simulink model "saturn_ib_stack_test"  (Simulink 6.2)
settings: Solver=ode4  SolverMode=SingleTasking  StartTime=-20.0  StopTime=620  FixedStep=0.005  RelTol=1e-3
values from neighbouring files (symbols this model uses):
  A_z_deg = 82.8200    (= 82.82)    [AS205_presettings.m]
  BN_1_sec = 14.4    [AS205_presettings.m]
  DeltaV_b_mps = 7.2381    [AS205_presettings.m]
  epsilon_2_sec = 15.0    (= 15)    [AS205_presettings.m]
  epsilon_prime_sec = 3.0    (= 3)    [AS205_presettings.m]
  i_deg = 28.89597    [AS205_presettings.m]
  lambda_0_deg = 102.32900    (= 102.329)    [AS205_presettings.m]
  lambda_L_deg = -80.561141    [AS205_presettings.m]
  pad_roll_L_deg = 100.0    (= 100)    [AS205_presettings.m]
  phi_L_deg = 28.521963    [AS205_presettings.m]
  phi_L_prime_deg = 28.360795    [AS205_presettings.m]
  R_L_m = 6373385.0    (= 6373385)    [AS205_presettings.m]
  R_T_m = 6570774.0    (= 6570774)    [AS205_presettings.m]
  T3_FM_sec = 6.08    [AS205_presettings.m]
  T_HSL_sec = 5.0    (= 5)    [AS205_presettings.m]
  Theta_T_deg = 0.000    (= 0)    [AS205_presettings.m]
  V_T_mps = 7780.976    [AS205_presettings.m]
  Xdotdot_VGT_mps2 = -9.251    [AS205_presettings.m]
undefined symbols (not defined in the file or in its folder): e0_0, e1_0, e2_0, e3_0, m, s
libraries: simulink x99, aerolibconvert x83, aerolibutil x63, aerolibtransform2 x34, aerolibasang x2, aerolibatmos2 x2, aerolib6dofsys x2
(part 5 of 7)

== system saturn_ib_stack_test/Saturn_IB_Stack/S-IVB Stage/APS III Module/APS Thruster II ==
  Fire : Inport  Port=1  LatchInput=off
  Cg_m : Inport  Port=2  PortDimensions=3  LatchInput=off
  3x3 Cross Product : aerolibutil/3x3 Cross Product
  Add : Sum  Inputs=+-  OutScaling=2^-10
  Constant2 : Constant  Value=[0.0 0.0 0.0]
  Installation location (m) : Constant  Value=r_m  OutDataTypeMode=double
  Switch : Switch  Criteria=u2 ~= 0
  Thruster Force : Constant  Value=F_N  OutDataTypeMode=double
  F_N : Outport
  M_Nm : Outport  Port=2
  wires:
  Cg_m/1 -> Add/2
  Installation location (m)/1 -> Add/1
  Add/1 -> 3x3 Cross Product/1
  3x3 Cross Product/1 -> M_Nm/1
  Switch/1 -> 3x3 Cross Product/2, F_N/1
  Thruster Force/1 -> Switch/1
  Constant2/1 -> Switch/3
  Fire/1 -> Switch/2

== system saturn_ib_stack_test/Saturn_IB_Stack/S-IVB Stage/APS III Module/APS Thruster IV ==
  Fire : Inport  Port=1  LatchInput=off
  Cg_m : Inport  Port=2  PortDimensions=3  LatchInput=off
  3x3 Cross Product : aerolibutil/3x3 Cross Product
  Add : Sum  Inputs=+-  OutScaling=2^-10
  Constant2 : Constant  Value=[0.0 0.0 0.0]
  Installation location (m) : Constant  Value=r_m  OutDataTypeMode=double
  Switch : Switch  Criteria=u2 ~= 0
  Thruster Force : Constant  Value=F_N  OutDataTypeMode=double
  F_N : Outport
  M_Nm : Outport  Port=2
  wires:
  Cg_m/1 -> Add/2
  Installation location (m)/1 -> Add/1
  Add/1 -> 3x3 Cross Product/1
  3x3 Cross Product/1 -> M_Nm/1
  Switch/1 -> 3x3 Cross Product/2, F_N/1
  Thruster Force/1 -> Switch/1
  Constant2/1 -> Switch/3
  Fire/1 -> Switch/2

== system saturn_ib_stack_test/Saturn_IB_Stack/S-IVB Stage/APS III Module/APS Thruster P ==
  Fire : Inport  Port=1  LatchInput=off
  Cg_m : Inport  Port=2  PortDimensions=3  LatchInput=off
  3x3 Cross Product : aerolibutil/3x3 Cross Product
  Add : Sum  Inputs=+-  OutScaling=2^-10
  Constant2 : Constant  Value=[0.0 0.0 0.0]
  Installation location (m) : Constant  Value=r_m  OutDataTypeMode=double
  Switch : Switch  Criteria=u2 ~= 0
  Thruster Force : Constant  Value=F_N  OutDataTypeMode=double
  F_N : Outport
  M_Nm : Outport  Port=2
  wires:
  Cg_m/1 -> Add/2
  Installation location (m)/1 -> Add/1
  Add/1 -> 3x3 Cross Product/1
  3x3 Cross Product/1 -> M_Nm/1
  Switch/1 -> 3x3 Cross Product/2, F_N/1
  Thruster Force/1 -> Switch/1
  Constant2/1 -> Switch/3
  Fire/1 -> Switch/2

== system saturn_ib_stack_test/Saturn_IB_Stack/S-IVB Stage/Custom Variable Mass 6DoF (Quaternion)/Calculate DCM & Euler Angles ==
  p q r : Inport  Port=1  LatchInput=off
  Initial quaternion : Inport  Port=2  LatchInput=off
  Quaternions to  Direction Cosine Matrix : aerolibtransform2/Quaternions to  Direction Cosine Matrix
  Quaternions to Euler Angles : aerolibtransform2/Quaternions to Euler Angles
  q0 q1 q2 q3 : Integrator  InitialConditionSource=external  InitialCondition=[e0_0 e1_0 e2_0 e3_0]
  qdot : Subsystem
  DCM : Outport
  Euler : Outport  Port=2
  q : Outport  Port=3
  wires:
  Quaternions to Euler Angles/1 -> Euler/1
  Quaternions to  Direction Cosine Matrix/1 -> DCM/1
  p q r/1 -> qdot/1(p q r)
  Initial quaternion/1 -> q0 q1 q2 q3/2
  q0 q1 q2 q3/1 -> Quaternions to  Direction Cosine Matrix/1, Quaternions to Euler Angles/1, qdot/2(q0 q1 q2 q3), q/1
  qdot/1(qdot) -> q0 q1 q2 q3/1

== system saturn_ib_stack_test/Saturn_IB_Stack/S-IVB Stage/Custom Variable Mass 6DoF (Quaternion)/Calculate omega_dot ==
  p q r : Inport  Port=1  LatchInput=off
  "I, I_dot" : Inport  Port=2  LatchInput=off
  Moments : Inport  Port=3  LatchInput=off
  I x w : Subsystem
  I x w1 : Subsystem
  Product2 : Product  Inputs=/*  Multiplication=Matrix(*)  SaturateOnIntegerOverflow=on
  Reshape : simulink/Math Operations/Reshape  OutputDimensionality=1-D array  OutputDimensions=[1,1]
  Selector : Selector  InputType=Matrix  Elements=[1 2 1]  Rows=1:3  Columns=-1  InputPortWidth=2
  Selector1 : Selector  InputType=Matrix  Elements=[1 2 1]  Rows=4:6  Columns=-1  InputPortWidth=2
  Selector2 : Selector  InputType=Matrix  Elements=[1 2 1]  Rows=1:3  Columns=-1  InputPortWidth=2
  Sum2 : Sum  Inputs=+--  SaturateOnIntegerOverflow=on
  wx(Iw) : aerolibutil/3x3 Cross Product
  pdot qdot rdot : Outport
  wires:
  I x w/1(I * w) -> wx(Iw)/2
  wx(Iw)/1 -> Sum2/3
  Selector1/1 -> I x w1/1(I_dot)
  I x w1/1(Id * w) -> Sum2/2
  Moments/1 -> Sum2/1
  Sum2/1 -> Product2/2
  Product2/1 -> Reshape/1
  p q r/1 -> I x w1/2(p q r), wx(Iw)/1, I x w/1(p q r)
  "I, I_dot"/1 -> Selector1/1, Selector2/1, Selector/1
  Selector2/1 -> Product2/1
  Selector/1 -> I x w/2(Inertia)
  Reshape/1 -> pdot qdot rdot/1

== system saturn_ib_stack_test/Saturn_IB_Stack/S-IVB Stage/Custom Variable Mass 6DoF (Quaternion)/transform to Inertial axes  ==
  x y z : Inport  Port=1  LatchInput=off
  transform coefficients : Inport  Port=2  LatchInput=off
  Product : Product  Multiplication=Matrix(*)  SaturateOnIntegerOverflow=on  InputSameDT=on
  Ve : Outport
  wires:
  Product/1 -> Ve/1
  transform coefficients/1 -> Product/1
  x y z/1 -> Product/2

== system saturn_ib_stack_test/Saturn_IB_Stack/S-IVB Stage/J-2 Engine/Thrust Model ==
  note: Mass flow rate prior to EMRC used here; 202.702 after EMRC
  note: STA 1086 of the full L/V stack
      | corresponds to STA 0.0 of the S-IVB
  Cg_m : Inport  Port=1  PortDimensions=3  LatchInput=off
  Pitch_actuator_cmd_deg : Inport  Port=2  PortDimensions=1  LatchInput=off
  Yaw_actuator_cmd_deg : Inport  Port=3  PortDimensions=1  LatchInput=off
  bEngineStart : Inport  Port=4  PortDimensions=1  DataType=boolean  LatchInput=off
  bEngineCutoff : Inport  Port=5  PortDimensions=1  DataType=boolean  LatchInput=off
  3x3 Cross Product : aerolibutil/3x3 Cross Product
  Add : Sum  Inputs=+-  OutScaling=2^-10
  Angle Conversion3 : aerolibconvert/Angle Conversion  IU=deg  OU=rad
  Bias : Bias  Bias=147.26
  Constant1 : Constant  Value=0.0
  Constant2 : Constant  Value=0.0
  Constant3 : Constant  Value=1010719
  Divide : Product  Inputs=**/  OutScaling=2^-10
  Euler Angles to  Direction Cosine Matrix3 : aerolibtransform2/Euler Angles to  Direction Cosine Matrix
  Gimbal Limits{,1..3} (4 alike) : Saturate  UpperLimit=7.0  LowerLimit=-7.0
  Installation location (in) : Constant  Value=[0.0 0.0 0.0]  OutDataTypeMode=double
  Mux : Mux  Inputs=3
  Mux1 : Mux  Inputs=3
  Pitch Actuator : TransferFcn  Denominator=[0.34542E-04 0.16582E-02 0.62686E-01 1.0]
  Product : Product  RndMeth=Zero
  Product3 : Product  Multiplication=Matrix(*)  RndMeth=Zero
  Thrust Decay : Lookup  InputValues=[0.0 0.2 0.3 0.5]  OutputValues=[1.0 0.05 0.03 0.0]  LookUpMeth=Interpolation-Use End Values
  Thrust vs. Time : Lookup  InputValues=|  OutputValues=|  LookUpMeth=Interpolation-Use End Values
      InputValues=|
      | [147.26
      | 148.58
      | 151.50
      | 151.98
      | 155.00
      | 159.18
      | 160.00
      | 180.00
      | 186.88
      | 190.00
      | 200.00
      | 220.00
      | 240.00
      | 260.00
      | 280.00
      | 300.00
      | 320.00
      | 340.00
      | 360.00
      | 380.00
      | 400.00
      | 420.00
      | 440.00
      | 460.00
      | 477.00
      | 480.00
      | 500.00
      | 520.00
      | 540.00
      | 560.00
      | 580.00
      | 592.91
      | ]
      OutputValues=|
      | [0
      | 0
      | 752069
      | 870634
      | 885366
      | 1010719
      | 1010474
      | 1009306
      | 1009198
      | 1009388
      | 1010028
      | 1007947
      | 1008703
      | 1009688
      | 1006171
      | 1008973
      | 1009424
      | 1008389
      | 1008991
      | 1007469
      | 1006695
      | 1009101
      | 1008642
      | 1005132
      | 958467
      | 940828
      | 873262
      | 859576
      | 847063
      | 847126
      | 852022
      | 850281
      | ]
  Time Since Engine Start : Subsystem
  Time Since Shutdown : Subsystem
  Unary Minus2 : simulink/Math Operations/Unary Minus  DoSatur=off
  Yaw Actuator : TransferFcn  Denominator=[0.34542E-04 0.16582E-02 0.62686E-01 1.0]
  in to m : Gain  Gain=0.0254
  m_dot : Constant  Value=243.687
  F_N : Outport
  M_Nm : Outport  Port=2
  mdot_kg_sec : Outport  Port=3
  wires:
  Cg_m/1 -> Add/2
  Installation location (in)/1 -> in to m/1
  Add/1 -> 3x3 Cross Product/1
  Pitch_actuator_cmd_deg/1 -> Gimbal Limits1/1
  Pitch Actuator/1 -> Gimbal Limits2/1
  Constant1/1 -> Mux/1
  Mux/1 -> Unary Minus2/1
  Angle Conversion3/1 -> Euler Angles to  Direction Cosine Matrix3/1
  Euler Angles to  Direction Cosine Matrix3/1 -> Product3/1
  Product3/1 -> 3x3 Cross Product/2, F_N/1
  Gimbal Limits/1 -> Yaw Actuator/1
  Gimbal Limits1/1 -> Pitch Actuator/1
  Yaw_actuator_cmd_deg/1 -> Gimbal Limits/1
  Mux1/1 -> Product3/2
  bEngineCutoff/1 -> Time Since Shutdown/1(bStart)
  Time Since Shutdown/1(T_elapsed_sec) -> Thrust Decay/1
  Constant2/1 -> Mux1/3, Mux1/2
  Time Since Engine Start/1(T_elapsed_sec) -> Bias/1
  bEngineStart/1 -> Time Since Engine Start/1(bStart)
  m_dot/1 -> Divide/1
  Divide/1 -> mdot_kg_sec/1
  Constant3/1 -> Divide/3
  Bias/1 -> Thrust vs. Time/1
  Yaw Actuator/1 -> Gimbal Limits3/1
  Gimbal Limits2/1 -> Mux/2
  Gimbal Limits3/1 -> Mux/3
  3x3 Cross Product/1 -> M_Nm/1
  in to m/1 -> Add/1
  Unary Minus2/1 -> Angle Conversion3/1
  Thrust vs. Time/1 -> Product/1
  Product/1 -> Mux1/1, Divide/2
  Thrust Decay/1 -> Product/2

== system saturn_ib_stack_test/Saturn_IB_Stack/S-IVB Stage/Relative Wind/Incidence, Sideslip, & Airspeed ==
  Vb : Inport  Port=1  LatchInput=off
  Airspeed : Math  Operator=sqrt  SaturateOnIntegerOverflow=on
  Compare To Zero : simulink/Logic and Bit Operations/Compare To Zero  relop=>  LogicOutDataTypeMode=boolean  ZeroCross=off
  Constant : Constant  Value=0.0
  Demux : Demux  Outputs=2
  Dot Product : simulink/Math Operations/Dot Product  InputSameDT=on  OutDataType=sfix(16)  OutScaling=2^-10  DoSatur=off
  Incidence : Trigonometry  Operator=atan2
  Product : Product  Inputs=*/  SaturateOnIntegerOverflow=on
  Selector : Selector  Elements=2  InputPortWidth=3
  Selector1 : Selector  Elements=[3 1]  InputPortWidth=3
  Sideslip : Trigonometry  Operator=asin
  Switch : Switch  Criteria=u2 ~= 0
  Alpha : Outport  InitialOutput=0
  Beta : Outport  Port=2  InitialOutput=0
  V : Outport  Port=3  InitialOutput=0
  wires:
  Product/1 -> Sideslip/1
  Demux/1 -> Incidence/1
  Demux/2 -> Incidence/2
  Selector1/1 -> Demux/1
  Dot Product/1 -> Airspeed/1
  Airspeed/1 -> V/1, Product/2, Compare To Zero/1
  Incidence/1 -> Alpha/1
  Vb/1 -> Selector1/1, Dot Product/1, Dot Product/2, Selector/1
  Selector/1 -> Product/1
  Compare To Zero/1 -> Switch/2
  Sideslip/1 -> Switch/1
  Switch/1 -> Beta/1
  Constant/1 -> Switch/3

== system saturn_ib_stack_test/Saturn_IB_Stack/S-IVB Stage/Ullage Rocket Motors/Time Since Engine Start ==
  bStart : Inport  Port=1  DataType=boolean  LatchInput=off
  Clock : Clock
      settings: Decimation=10
  Constant : Constant  Value=0.0
  Data Store Memory : DataStoreMemory  DataStoreName=A  InitialValue=-1  DataType=double
  Data Store Read : DataStoreRead  DataStoreName=A  SampleTime=0
  Sum : Sum  Inputs=|+-
  Switch : Switch  Threshold=0.0
  Timer Initialization : Subsystem  TreatAsAtomicUnit=on
  T_elapsed_sec : Outport
  wires:
  bStart/1 -> Timer Initialization/Trigger
  Clock/1 -> Timer Initialization/1(In1), Sum/1
  Switch/1 -> T_elapsed_sec/1
  Sum/1 -> Switch/1
  Data Store Read/1 -> Sum/2, Switch/2
  Constant/1 -> Switch/3

== system saturn_ib_stack_test/Saturn_IB_Stack/Saturn Instrument Unit (IU)/Flight Control Computer/S-IB Attitude Error Filters ==
  In1 : Inport  Port=1  LatchInput=off
  Demux1 : Demux  Outputs=3
  Mux3 : Mux  Inputs=3
  Transfer Fcn3 : TransferFcn  Denominator=[0.1584 1]
  Transfer Fcn4 : TransferFcn  Denominator=[0.1320 1]
  Transfer Fcn5 : TransferFcn  Denominator=[0.1320 1]
  Out1 : Outport
  wires:
  Demux1/2 -> Transfer Fcn4/1
  Demux1/1 -> Transfer Fcn3/1
  Transfer Fcn3/1 -> Mux3/1
  Transfer Fcn4/1 -> Mux3/2
  Demux1/3 -> Transfer Fcn5/1
  Transfer Fcn5/1 -> Mux3/3
  In1/1 -> Demux1/1
  Mux3/1 -> Out1/1

== system saturn_ib_stack_test/Saturn_IB_Stack/Saturn Instrument Unit (IU)/Flight Control Computer/S-IB Attitude Rate Error ==
  In1 : Inport  Port=1  LatchInput=off
  Demux : Demux  Outputs=3
  Ground : Ground
  Mux2 : Mux  Inputs=3
  Terminator : Terminator
  Transfer Fcn : TransferFcn  Numerator=[0.0021 0.012 1]  Denominator=[0.0006193 0.01358 0.1597 1]
  Transfer Fcn1 : TransferFcn  Numerator=[0.0003640 0.001040 1]  Denominator=[0.0000668 0.01650 0.1560 1]
  Transfer Fcn2 : TransferFcn  Numerator=[0.0003640 0.001040 1]  Denominator=[0.0000668 0.01650 0.1560 1]
  Out1 : Outport
  wires:
  Transfer Fcn2/1 -> Mux2/3
  Demux/3 -> Transfer Fcn2/1
  Demux/2 -> Transfer Fcn1/1
  Transfer Fcn1/1 -> Mux2/2
  Demux/1 -> Transfer Fcn/1
  Transfer Fcn/1 -> Mux2/1
  In1/1 -> Out1/1
  Ground/1 -> Demux/1
  Mux2/1 -> Terminator/1

== system saturn_ib_stack_test/Saturn_IB_Stack/Saturn Instrument Unit (IU)/Flight Control Computer/S-IB Y/Z Acceleration Filters ==
  In1 : Inport  Port=1  LatchInput=off
  Demux2 : Demux  Outputs=3
  Mux4 : Mux  Inputs=3
  Transfer Fcn6 : TransferFcn  Denominator=[0.5 5.1 1.0]
  Transfer Fcn7 : TransferFcn  Denominator=[0.5 5.1 1.0]
  Out1 : Outport
  wires:
  Demux2/2 -> Transfer Fcn7/1
  Demux2/1 -> Mux4/1
  Transfer Fcn7/1 -> Mux4/2
  Demux2/3 -> Transfer Fcn6/1
  Transfer Fcn6/1 -> Mux4/3
  In1/1 -> Demux2/1
  Mux4/1 -> Out1/1

== system saturn_ib_stack_test/Saturn_IB_Stack/Saturn Instrument Unit (IU)/Flight Control Computer/S-IVB Pitch/Yaw Attitude Rate Filters ==
  In1 : Inport  Port=1  LatchInput=off
  bSwitchpoint5 : Inport  Port=2  LatchInput=off
  Demux1 : Demux  Outputs=3
  Demux4 : Demux  Outputs=3
  Logical Operator : Logic  Operator=NOT  AllPortsSameDT=off  OutDataTypeMode=Boolean
  Mux1 : Mux  Inputs=3
  Mux10 : Mux  Inputs=3
  Switch : Switch  Criteria=u2 ~= 0
  Transfer Fcn1 : TransferFcn  Numerator=[0.14e-03 0.4e-03 1]  Denominator=[0.7462e-04 0.3842e-02 0.7974e-01 1]
  Transfer Fcn10 : TransferFcn  Numerator=[0.14e-03 0.4e-3 1]  Denominator=[0.7225e-4 0.3759e-2 0.7917e-01 1]
  Transfer Fcn11 : TransferFcn  Numerator=[0.14e-03 0.4e-3 1]  Denominator=[0.7225e-4 0.3759e-2 0.7917e-01 1]
  Transfer Fcn2 : TransferFcn  Numerator=[0.14e-03 0.4e-03 1]  Denominator=[0.7462e-04 0.3842e-02 0.7974e-01 1]
  Out1 : Outport
  wires:
  Demux4/1 -> Mux10/1
  Transfer Fcn11/1 -> Mux10/2
  Demux4/2 -> Transfer Fcn11/1
  Demux4/3 -> Transfer Fcn10/1
  Transfer Fcn10/1 -> Mux10/3
  Mux10/1 -> Switch/1
  Logical Operator/1 -> Switch/2
  bSwitchpoint5/1 -> Logical Operator/1
  Demux1/1 -> Mux1/1
  Transfer Fcn2/1 -> Mux1/2
  Demux1/2 -> Transfer Fcn2/1
  Demux1/3 -> Transfer Fcn1/1
  Transfer Fcn1/1 -> Mux1/3
  Mux1/1 -> Switch/3
  Switch/1 -> Out1/1
  In1/1 -> Demux4/1, Demux1/1

== system saturn_ib_stack_test/Saturn_IB_Stack/Saturn Instrument Unit (IU)/Flight Control Computer/S-IVB Pitch/Yaw  Attitude Error Filters ==
  In1 : Inport  Port=1  LatchInput=off
  bSwitchpoint5 : Inport  Port=2  LatchInput=off
  Demux1 : Demux  Outputs=3
  Demux3 : Demux  Outputs=3
  Logical Operator : Logic  Operator=NOT  AllPortsSameDT=off  OutDataTypeMode=Boolean
  Mux1 : Mux  Inputs=3
  Mux9 : Mux  Inputs=3
  Switch : Switch  Criteria=u2 ~= 0
  Transfer Fcn1 : TransferFcn  Denominator=[0.1556 1]
  Transfer Fcn2 : TransferFcn  Denominator=[0.1556 1]
  Transfer Fcn8 : TransferFcn  Denominator=[0.1545 1]
  Transfer Fcn9 : TransferFcn  Denominator=[0.1545 1]
  Out1 : Outport
  wires:
  Demux3/2 -> Transfer Fcn8/1
  Demux3/1 -> Mux9/1
  Transfer Fcn8/1 -> Mux9/2
  Demux3/3 -> Transfer Fcn9/1
  Transfer Fcn9/1 -> Mux9/3
  Demux1/2 -> Transfer Fcn1/1
  Demux1/1 -> Mux1/1
  Transfer Fcn1/1 -> Mux1/2
  Demux1/3 -> Transfer Fcn2/1
  Transfer Fcn2/1 -> Mux1/3
  Mux9/1 -> Switch/1
  Logical Operator/1 -> Switch/2
  bSwitchpoint5/1 -> Logical Operator/1
  Mux1/1 -> Switch/3
  Switch/1 -> Out1/1
  In1/1 -> Demux3/1, Demux1/1

== system saturn_ib_stack_test/Saturn_IB_Stack/Saturn Instrument Unit (IU)/Flight Control Computer/S-IVB Stage Timer ==
  bStart : Inport  Port=1  DataType=boolean  LatchInput=off
  Clock : Clock
      settings: Decimation=10
  Constant : Constant  Value=0.0
  Data Store Memory : DataStoreMemory  DataStoreName=A  InitialValue=-1  DataType=double
  Data Store Read : DataStoreRead  DataStoreName=A  SampleTime=0
  Sum : Sum  Inputs=|+-
  Switch : Switch  Threshold=0.0
  Timer Initialization : Subsystem  TreatAsAtomicUnit=on
  T_elapsed_sec : Outport
  wires:
  bStart/1 -> Timer Initialization/Trigger
  Clock/1 -> Timer Initialization/1(In1), Sum/1
  Switch/1 -> T_elapsed_sec/1
  Sum/1 -> Switch/1
  Data Store Read/1 -> Sum/2, Switch/2
  Constant/1 -> Switch/3

== system saturn_ib_stack_test/Saturn_IB_Stack/Saturn Instrument Unit (IU)/Flight Control Computer/Spatial Attitude Control System ==
  note: +P
  note: -P
  note: +Y - R
  note: -Y + R
  note: +Y +R
  note: -Y -R
  note: Based on Figure 3.4-3 from Astrionics System Handbook and
      | "S-IVB Polarity Table" from section 3-1 (NASA-CR-71607)
  note: Attitude error limits from
      | SLV, AS-205, Rev A
  AttitudeError_deg : Inport  Port=1  LatchInput=off
  AttitudeRate_deg_per_sec : Inport  Port=2  LatchInput=off
  bS_IVB_Burn : Inport  Port=3  LatchInput=off
  Constant : Constant  Value=0.0
  Demux : Demux  Outputs=3
  Demux1 : Demux  Outputs=3
  Derived Rate Modulator : Subsystem
  Derived Rate Modulator (Pitch) : Subsystem
  Derived Rate Modulator1 : Subsystem
  Gain : Gain  Gain=5.0
  Saturation : Saturate  UpperLimit=2.5  LowerLimit=-2.5
  Saturation1 : Saturate  UpperLimit=3.5  LowerLimit=-3.5
  Saturation2 : Saturate  UpperLimit=2.5  LowerLimit=-2.5
  Sum1 : Sum  Inputs=|+-
  Sum14 : Sum  Inputs=|++
  Sum2 : Sum  Inputs=++|
  Sum3 : Sum  Inputs=++|
  Sum4 : Sum  Inputs=|++
  Switch{,1..3} (4 alike) : Switch  Criteria=u2 ~= 0
  APS_III_P : Outport
  APS_III_II : Outport  Port=2
  APS_III_IV : Outport  Port=3
  APS_I_P : Outport  Port=4
  APS_I_II : Outport  Port=5
  APS_I_IV : Outport  Port=6
  wires:
  Sum3/1 -> Sum1/1, Sum2/2
  AttitudeError_deg/1 -> Demux/1
  AttitudeRate_deg_per_sec/1 -> Gain/1
  Saturation1/1 -> Sum14/1
  Saturation2/1 -> Sum3/2
  Demux/1 -> Saturation1/1
  Saturation/1 -> Sum4/1
  Sum4/1 -> Derived Rate Modulator (Pitch)/1(In)
  Demux1/1 -> Sum14/2
  Sum1/1 -> Derived Rate Modulator/1(In)
  Sum2/1 -> Derived Rate Modulator1/1(In)
  bS_IVB_Burn/1 -> Switch/2, Switch3/2, Switch1/2, Switch2/2
  Derived Rate Modulator (Pitch)/1(A) -> APS_I_P/1
  Derived Rate Modulator (Pitch)/2(B) -> APS_III_P/1
  Derived Rate Modulator1/1(A) -> APS_I_II/1
  Derived Rate Modulator/1(A) -> APS_III_II/1
  Derived Rate Modulator1/2(B) -> APS_I_IV/1
  Derived Rate Modulator/2(B) -> APS_III_IV/1
  Switch/1 -> Saturation2/1
  Switch1/1 -> Saturation/1
  Demux/2 -> Switch1/3
  Demux/3 -> Switch/3
  Gain/1 -> Demux1/1
  Sum14/1 -> Sum1/2, Sum2/1
  Switch3/1 -> Sum3/1
  Switch2/1 -> Sum4/2
  Demux1/2 -> Switch2/3
  Demux1/3 -> Switch3/3
  Constant/1 -> Switch2/1, Switch1/1, Switch3/1, Switch/1

== system saturn_ib_stack_test/Saturn_IB_Stack/Saturn Instrument Unit (IU)/LVDA / LVDC/LVDC Chi command angles (Time Tilt) ==
  note: Time Tilt equations from "AS-205 Revised L/V Reference Trajectory"
  T_c_sec : Inport  Port=1  SampleTime=0.04  LatchInput=off
  theta_x_deg : Inport  Port=2  LatchInput=off
  0 - T_S2 : Saturate  UpperLimit=137.0  LowerLimit=10.0  SampleTime=0.04
  Angle Conversion : aerolibconvert/Angle Conversion  IU=rad  OU=deg
  Compare To Constant : simulink/Logic and Bit Operations/Compare To Constant  relop=<=  const=10.0  LogicOutDataTypeMode=boolean  ZeroCross=off
  Data Store Read : DataStoreRead  DataStoreName=Chi_X_deg  SampleTime=0.04
  Data Store Read1 : DataStoreRead  DataStoreName=Chi_Y_deg  SampleTime=0.04
  Data Store Read2 : DataStoreRead  DataStoreName=Chi_Z_deg  SampleTime=0.04
  F_1 : simulink/Math Operations/Polynomial  coefs="[0.321123e-6   -0.165429e-3   0.284092e-02   -0.155517e-1  ]"
  F_2 : simulink/Math Operations/Polynomial  coefs=[0.101124e-5 -0.202467e-3 0.229458e-02 0.207839e-01]
  F_3 : simulink/Math Operations/Polynomial  coefs="[-0.997002e-6 0.337240e-03 -0.457693e-1   0.143848e01 ]"
  Mux : Mux  Inputs=3
  Mux1 : Mux  Inputs=3
  P_final : Constant  Value=-1.061769
  Rate Limiter Dynamic : Subsystem  AncestorBlock=simulink/Discontinuities/Rate Limiter Dynamic
      mask Type: Rate Limiter Dynamic
      mask Description: Limit rising and falling rates of the signals at the second input by using the first input (upper limit) and the third input (lower limit).
      mask Display: plot([0.15 0.95],[.5 .5],[.5 .5],[0.05 0.95],0.05+0.9*[.2 .8],0.05+0.9*[0 1]);
  Relational Operator{,1..3} (4 alike) : RelationalOperator  Operator=<=  LogicOutDataTypeMode=Boolean
  Store Chi Command Angles : Subsystem  TreatAsAtomicUnit=on
  Switch{,1..3,5} (5 alike) : Switch  Criteria=u2 ~= 0
  T_S1_sec : Constant  Value=45.0
  T_S1_sec1 : Constant  Value=10.0
  T_S2_sec : Constant  Value=92.0
  T_S3_sec : Constant  Value=137.0
  Unary Minus : simulink/Math Operations/Unary Minus  DoSatur=off
  chi rate limit : Constant  Value=[1 1 1]
  yaw command : Constant  Value=0.0
  zero : Constant  Value=0.0
  Chi_deg : Outport
  wires:
  T_c_sec/1 -> 0 - T_S2/1, Compare To Constant/1, Relational Operator3/1, Relational Operator2/1, Relational Operator1/1, Relational Operator/1
  Relational Operator/1 -> Switch/2
  T_S1_sec/1 -> Relational Operator/2
  Relational Operator1/1 -> Switch1/2
  F_2/1 -> Switch1/1
  Switch1/1 -> Switch/3
  T_S2_sec/1 -> Relational Operator1/2
  Relational Operator2/1 -> Switch2/2, Store Chi Command Angles/Enable
  F_3/1 -> Switch2/1
  T_S3_sec/1 -> Relational Operator2/2
  Switch2/1 -> Switch1/3
  0 - T_S2/1 -> F_3/1, F_2/1, F_1/1
  Switch3/1 -> Mux/1
  Compare To Constant/1 -> Switch3/2
  theta_x_deg/1 -> Switch3/1
  zero/1 -> Switch3/3, Switch5/1
  F_1/1 -> Switch/1
  T_S1_sec1/1 -> Relational Operator3/2
  Relational Operator3/1 -> Switch5/2
  Unary Minus/1 -> Rate Limiter Dynamic/3(lo)
  chi rate limit/1 -> Unary Minus/1, Rate Limiter Dynamic/1(up)
  yaw command/1 -> Mux/3
  Angle Conversion/1 -> Mux/2
  Switch5/1 -> Angle Conversion/1
  Switch/1 -> Switch5/3
  P_final/1 -> Switch2/3
  Rate Limiter Dynamic/1(Y) -> Chi_deg/1
  Mux1/1 -> Rate Limiter Dynamic/2(u)
  Data Store Read/1 -> Mux1/1
  Data Store Read1/1 -> Mux1/2
  Data Store Read2/1 -> Mux1/3
  Mux/1 -> Store Chi Command Angles/1(In1)

== system saturn_ib_stack_test/Saturn_IB_Stack/Saturn Instrument Unit (IU)/LVDA / LVDC/LVDC Chi to Psi Transformation ==
  note: Eqn 8.3.4
  note: Eqn 8.3.3
  note: Eqn 8.2.2
  Theta_deg : Inport  Port=1  SampleTime=0.04  LatchInput=off
  Chi_deg : Inport  Port=2  LatchInput=off
  Angle Conversion2 : aerolibconvert/Angle Conversion  IU=deg  OU=rad
  Demux : Demux  Outputs=3
  Demux1 : Demux  Outputs=2
  Demux2 : Demux  Outputs=2
  Gain1 : Gain  Gain=0.5
  Mux : Mux  Inputs=3
  Product{5..8,10} (5 alike) : Product  SampleTime=0.04  RndMeth=Zero
  Product3 : Product  RndMeth=Zero
  Product4 : Product  RndMeth=Zero
  Selector : Selector  Elements=[3 1]  InputPortWidth=3
  SinCos : aerolibutil/SinCos
  Sum1 : Sum  Inputs=|-+  SampleTime=0.04
  Sum2 : Sum  Inputs=++|  SampleTime=0.04
  Sum3 : Sum  Inputs=|++
  Sum4 : Sum  Inputs=|+-
  Sum5 : Sum  Inputs=|++
  Psi_deg : Outport
  wires:
  Chi_deg/1 -> Sum2/2, Sum1/1
  Sum4/1 -> Mux/3  "Psi_Y"
  Sum3/1 -> Mux/2  "Psi_P"
  SinCos/1 -> Demux1/1
  Sum5/1 -> Mux/1  "Psi_R"
  Selector/1 -> Gain1/1
  Sum2/1 -> Angle Conversion2/1
  Product10/1 -> Sum5/2
  Product8/1 -> Sum4/2
  Product7/1 -> Sum4/1
  Product6/1 -> Sum3/2
  Product5/1 -> Sum3/1
  Product4/1 -> Product8/1  "A4"
  Demux1/1 -> Product10/1  "A3"
  Demux1/2 -> Product4/1, Product6/1  "A2"
  Product3/1 -> Product5/1  "A1"
  Demux2/2 -> Product3/2, Product7/1  "A5"
  Demux2/1 -> Product3/1, Product4/2
  SinCos/2 -> Demux2/1
  Sum1/1 -> Demux/1  "delta Theta"
  Angle Conversion2/1 -> Selector/1
  Theta_deg/1 -> Sum2/1, Sum1/2
  Mux/1 -> Psi_deg/1  "Psi_deg"
  Gain1/1 -> SinCos/1
  Demux/1 -> Sum5/1
  Demux/2 -> Product10/2, Product5/2, Product8/2
  Demux/3 -> Product6/2, Product7/2

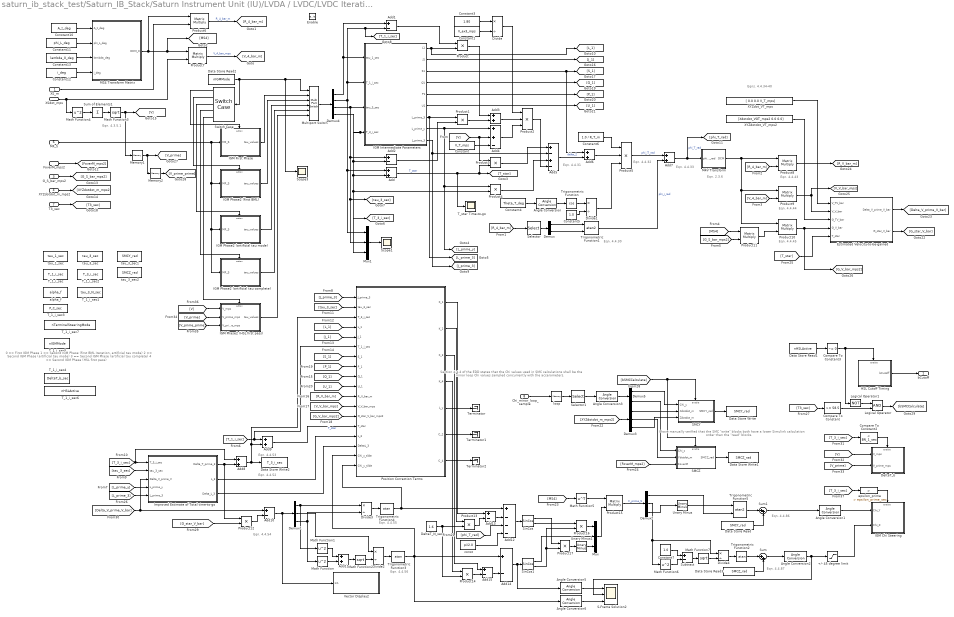
== system saturn_ib_stack_test/Saturn_IB_Stack/Saturn Instrument Unit (IU)/LVDA / LVDC/LVDC Iterative Guidance Mode ==
  note: Eqn. 4.4.31
  note: Eqn. 4.4.32
  note: Eqn. 4.4.33
  note: Eqn. 4.4.30
  note: Eqn. 2.3.6
  note: Eqn. 4.4.43
  note: Eqn. 4.4.44
  note: Eqn. 4.4.45
  note: Eqns. 4.4.34-40
  note: Eqn. 4.4.52
  note: Eqn. 4.4.53
  note: Eqn. 4.4.54
  note: Eqn. 4.4.55
  note: Eqn. 4.4.56
  note: 0 == First IGM Phase
      | 1 == Second IGM Phase (first BML iteration, artificial tau mode)
      | 2 == Second IGM Phase (artificial tau mode)
      | 3 == Second IGM Phase (artificial tau complete)
      | 4 == Second IGM Phase (HSL first pass)
  note: Eqn. 4.3.5.1
  note: Section 4.4.4 of the EDD states that
      | the Chi values used in SMC calculations shall be
      | the minor loop Chi values sampled concurrently
      | with the accerometers.
  note: I have manually verified that the
      | SMC "write" blocks both have a lower
      | Simulink calculation order than the
      | "read" blocks.
  note: Eqn. 4.4.86
  note: Eqn. 4.4.87
  XS_m : Inport  Port=1  PortDimensions=3  SampleTime=1.6  DataType=double  LatchInput=off
  XSdot_mps : Inport  Port=2  PortDimensions=3  SampleTime=1.6  DataType=double  LatchInput=off
  G_S_bar_mps2 : Inport  Port=3  PortDimensions=3  DataType=double  LatchInput=off
  XYZdotdot_m_mps2 : Inport  Port=4  PortDimensions=3  DataType=double  LatchInput=off
  FoverM_mps2 : Inport  Port=5  PortDimensions=1  SampleTime=1.6  DataType=double  LatchInput=off
  MF_S : Inport  Port=6  PortDimensions=1  SampleTime=1.6  DataType=double  LatchInput=off
  T3_sec : Inport  Port=7  PortDimensions=1  SampleTime=1.6  DataType=double  LatchInput=off
  Chi_minor_loop_sample : Inport  Port=8  PortDimensions=3  SampleTime=1.6  DataType=double  LatchInput=off
  Enable : EnablePort
  +/- 45 degree limit : Saturate  UpperLimit=45.0  LowerLimit=-45.0
  Add{,3,6,8..9,11} (6 alike) : Sum  OutScaling=2^-10
  Add{1..2,10,13..15} (6 alike) : Sum  Inputs=+-  OutScaling=2^-10
  Add12 : Sum  Inputs=+---  OutScaling=2^-10
  Add4 : Sum  Inputs=++-  OutScaling=2^-10
  Add5 : Sum  Inputs=+-+-  OutScaling=2^-10
  Add7 : Sum  OutScaling=2^-10  SampleTime=1.6
  Angle Conversion : aerolibconvert/Angle Conversion  IU=deg  OU=rad
  Angle Conversion{1..2,5..6} (4 alike) : aerolibconvert/Angle Conversion  IU=rad  OU=deg
  Angle Conversion3 : aerolibconvert/Angle Conversion  IU=deg  OU=rad
  Compare To Constant : simulink/Logic and Bit Operations/Compare To Constant  relop=>=  const=58.5  LogicOutDataTypeMode=uint8  ZeroCross=off
  Compare To Constant2 : simulink/Logic and Bit Operations/Compare To Constant  relop=<  const=BN_1_sec  LogicOutDataTypeMode=boolean  ZeroCross=off
  Compare To Constant3 : simulink/Logic and Bit Operations/Compare To Constant  relop=~=  const=0  LogicOutDataTypeMode=boolean  ZeroCross=off
  Constant : Constant  Value=V_T_mps
  Constant1 : Constant  Value=V_ex3_mps
  Constant10 : Constant  Value=A_z_deg
  Constant11 : Constant  Value=phi_L_deg
  Constant12 : Constant  Value=i_deg
  Constant13 : Constant  Value=lambda_0_deg
  Constant3 : Constant  Value=1.80
  Constant4 : Constant  Value=Theta_T_deg
  Constant5 : Constant  Value=1.0
  Constant6 : Constant  Value=1.0 / R_T_m
  Constant7 : Constant  Value=1.0
  Data Store Read : DataStoreRead  DataStoreName=SMCY_rad  SampleTime=1.6
  Data Store Read1 : DataStoreRead  DataStoreName=nHSLActive  SampleTime=0.04
  Data Store Read2 : DataStoreRead  DataStoreName=nIGMMode  SampleTime=1.6
  Data Store Read3 : DataStoreRead  DataStoreName=SMCZ_rad  SampleTime=1.6
  Data Store Write : DataStoreWrite  DataStoreName=SMCY_rad  SampleTime=-1
  Data Store Write1 : DataStoreWrite  DataStoreName=SMCZ_rad  SampleTime=-1
  Data Store Write2 : DataStoreWrite  DataStoreName=T_3_i_sec  SampleTime=-1
  DeltaT_N_sec : Constant  Value=1.6
  DeltaT_b : Subsystem  TreatAsAtomicUnit=on
  Demux : Demux  Outputs=2
  Demux1 : Demux  Outputs=3
  Demux2 : Demux  Outputs=3
  Demux3 : Demux  Outputs=3
  Demux4 : Demux
  Demux5 : Demux  Outputs=2
  Divide{,1..4} (5 alike) : Product  Inputs=*/  OutScaling=2^-10
  Estimated Velocity-to-be-gained : Subsystem
  HSL Cutoff Timing : Subsystem  TreatAsAtomicUnit=on
  IGM Chi Steering : Subsystem  TreatAsAtomicUnit=on
  IGM First Phase : Subsystem  TreatAsAtomicUnit=on
  IGM Intermediate Parameters : Subsystem
  IGM Phase2 (HSL first pass) : Subsystem  TreatAsAtomicUnit=on
  IGM Phase2 (artificial tau complete) : Subsystem  TreatAsAtomicUnit=on
  IGM Phase2 (artificial tau mode) : Subsystem  TreatAsAtomicUnit=on
  IGM Phase2 (first BML) : Subsystem  TreatAsAtomicUnit=on
  Improved Estimate of Total time-to-go : Subsystem
  Logical Operator : Logic  AllPortsSameDT=off  OutDataTypeMode=Boolean
  Logical Operator1 : Logic  Operator=NOT  AllPortsSameDT=off  OutDataTypeMode=Boolean  SampleTime=1.6
  M4V Transform : Subsystem  AncestorBlock="aerolibtransform2/Euler Angles to  Direction Cosine Matrix"
      mask Type: Euler2DCM
      mask Description: M4V transformation DCM
      mask Display: disp('M4V')
  MS4 Transform Matrix : Subsystem  TreatAsAtomicUnit=on
  Math Function{,1,4,6} (4 alike) : Math  Operator=square  SaturateOnIntegerOverflow=on
  Math Function2 : Math  Operator=sqrt  SaturateOnIntegerOverflow=on
  Math Function3 : Math  Operator=sqrt  SaturateOnIntegerOverflow=on
  Math Function5 : Math  Operator=transpose  SaturateOnIntegerOverflow=on
  Math Function7 : Math  Operator=sqrt  SaturateOnIntegerOverflow=on
  Memory1 : Memory  InheritSampleTime=on
  Memory2 : Memory  InheritSampleTime=on
  Multiport Switch : MultiPortSwitch  Inputs=5  zeroidx=on
  Mux : Mux  Inputs=3
  Mux1 : Mux  Inputs=3
  Position Correction Terms : Subsystem  TreatAsAtomicUnit=on  SystemSampleTime=1.6
  Product{,1,3..4,12..14,16..17} (9 alike) : Product  RndMeth=Zero
  Product{6..11,15} (7 alike) : Product  Multiplication=Matrix(*)  RndMeth=Zero
  Product2 : Product  Inputs=3  RndMeth=Zero
  Product5 : Product  Inputs=3  RndMeth=Zero
  S-Frame Solution2 : Scope  NumInputPorts=3
      settings: TimeRange=400  YMin=-0.065~2.43~0  YMax=-0.058~2.49~1  SaveName=ScopeData35
  SMCY : Subsystem
  SMCZ : Subsystem
  Scope1 : Scope
      settings: YMin=0  YMax=325  SaveName=ScopeData10
  Scope3 : Scope
      settings: YMin=2.85  YMax=3.15  SaveName=ScopeData13
  Selector : Selector  Elements=[3 1]  InputPortWidth=3
  Selector1 : Selector  Elements=[2 3]  InputPortWidth=3
  SinCos : aerolibutil/SinCos
  SinCos1 : aerolibutil/SinCos
  Subtract : Sum  Inputs=+-  OutScaling=2^-10
  Sum : Sum  Inputs=|++  SampleTime=1.6
  Sum of Elements1 : Sum  Inputs=+  OutScaling=2^-10
  Sum1 : Sum  Inputs=|++  SampleTime=1.6
  Switch Case : SwitchCase  Orientation=left  CaseConditions={0,1,2,3,4}  CaseShowDefault=off  SampleTime=1.6
  T_1_i_sec : DataStoreMemory  DataStoreName=T_1_i_sec  InitialValue=tau_1_i_preset_sec  DataType=double
  T_1_i_sec1 : DataStoreMemory  DataStoreName=tau_3_N_sec  InitialValue=tau_1_i_preset_sec  DataType=double
  T_1_i_sec2 : DataStoreMemory  DataStoreName=T_3_i_sec  InitialValue=tau_3_i_preset_sec  DataType=double
  T_1_i_sec3 : DataStoreMemory  DataStoreName=P_C_sec  InitialValue=0.0  DataType=double
  T_1_i_sec4 : DataStoreMemory  DataStoreName=DeltaT_b_sec  InitialValue=0.0  DataType=double
  T_1_i_sec5 : DataStoreMemory  DataStoreName=nIGMMode  InitialValue=0  DataType=int8
  T_1_i_sec6 : DataStoreMemory  DataStoreName=nHSLActive  InitialValue=0  DataType=int32
  T_1_i_sec7 : DataStoreMemory  DataStoreName=nTerminalSteeringMode  InitialValue=0  DataType=int8
  T_star Time-to-go : Scope
      settings: YMin=230  YMax=325  SaveName=ScopeData14
  Terminator : Terminator
  Terminator1 : Terminator
  Terminator2 : Terminator
  Trigonometric Function : Trigonometry  Operator=cos
  Trigonometric Function1 : Trigonometry  Operator=atan2
  Trigonometric Function2 : Trigonometry  Operator=atan
  Trigonometric Function3 : Trigonometry  Operator=atan
  Trigonometric Function4 : Trigonometry  Operator=atan
  Trigonometric Function5 : Trigonometry  Operator=atan2
  Unary Minus : simulink/Math Operations/Unary Minus  DoSatur=off
  Unary Minus1 : simulink/Math Operations/Unary Minus  DoSatur=off
  Vector Display2 : Subsystem
  XYZdot_VT_mps : Constant  Value=[ 0.0 0.0 V_T_mps]  SampleTime=1.6
  XYZdotdot_VT_mps2 : Constant  Value=[Xdotdot_VGT_mps2 0.0 0.0]  SampleTime=1.6
  alpha_f : DataStoreMemory  DataStoreName=alpha_f  InitialValue=tau_1_i_preset_sec  DataType=double
  const : Constant  Value=pi/2.0
  epsilon_prime : simulink/Logic and Bit Operations/Compare To Constant  relop=>  const=epsilon_prime_sec  LogicOutDataTypeMode=boolean  ZeroCross=off
  loop : Memory  InheritSampleTime=on
  tau_1_sec : DataStoreMemory  DataStoreName=tau_1_sec  InitialValue=T10_sec  DataType=double
  tau_3_sec : DataStoreMemory  DataStoreName=tau_3_sec  InitialValue=tau_3_preset_sec  DataType=double
  tau_3_sec1 : DataStoreMemory  DataStoreName=SMCY_rad  InitialValue=0.0  DataType=double
  tau_3_sec2 : DataStoreMemory  DataStoreName=SMCZ_rad  InitialValue=0.0  DataType=double
  bCutoff : Outport  PortDimensions=1  SampleTime=0.04  DataType=boolean  InitialOutput=[false]
  wires:
  FoverM_mps2/1 -> [FoverM_mps2]
  Demux4/2 -> Add1/2, [T_1_i_sec], IGM Intermediate Parameters/2(T_1_i_sec), Add/1, Mux1/1
  Demux4/3 -> IGM Intermediate Parameters/3(tau_3_sec), Add2/1, [tau_3_sec], Mux1/2
  Demux4/4 -> Add/2, Product4/2, [T_3_i_sec], IGM Intermediate Parameters/4(T_3_i_sec), Add2/2, Mux1/3
  Add/1 -> Product3/2, [T_star], T_star Time-to-go/1  "T_star"
  IGM Intermediate Parameters/1(L1) -> Product/2, [L_1]
  Add1/1 -> Product/1
  IGM Intermediate Parameters/7(L_prime_3) -> Product1/1, [L_prime_3]
  Add2/1 -> Product1/2
  Product/1 -> Add3/1
  Product1/1 -> Add3/2
  IGM Intermediate Parameters/8(L_prime_y) -> Add4/1, Product4/1, [L_prime_y]
  Add3/1 -> Product2/2
  Add4/1 -> Product2/3
  Constant/1 -> Add4/3
  Add5/1 -> Add6/2  "delta_2"
  Product3/1 -> Add5/1
  IGM Intermediate Parameters/9(J_prime_3) -> Add5/2, [J_prime_3]
  Product4/1 -> Add5/3
  Divide/1 -> Product2/1
  Constant1/1 -> Divide/2
  Constant3/1 -> Divide/1
  [V] -> Add4/2, Product3/1
  IGM Intermediate Parameters/3(S1) -> [S_1], Add6/1
  Trigonometric Function/1 -> Divide1/1
  Angle Conversion/1 -> Trigonometric Function/1
  Constant4/1 -> Angle Conversion/1
  Constant5/1 -> Divide1/2
  Divide1/1 -> Product5/3
  Add6/1 -> Product5/2
  Constant6/1 -> Product5/1
  Product5/1 -> Add7/1  "phi_iT_rad"
  Trigonometric Function1/1 -> Add7/2  "phi_i_rad"
  Add7/1 -> M4V Transform/1(phi_T_rad), [phi_T_rad]  "phi_T_rad"
  Demux/1 -> Trigonometric Function1/1
  Demux/2 -> Trigonometric Function1/2
  MS4 Transform Matrix/1(DCM_0) -> Product6/1, [MS4], Product7/1
  XS_m/1 -> Product6/2
  XSdot_mps/1 -> Math Function4/1, Product7/2
  Product7/1 -> [V_4_bar_m]  "V_4_bar_mps"
  Product6/1 -> [R_4_bar_m]  "R_4_bar_m"
  [R_4_bar_m] -> Selector/1
  Selector/1 -> Demux/1
  M4V Transform/1(DCM) -> Product8/1, Product9/1, Product10/1
  [R_4_bar_m] -> Product8/2
  [V_4_bar_m] -> Product9/2
  Product11/1 -> Product10/2
  [MS4] -> Product11/1
  [G_S_bar_mps2] -> Product11/2
  Product10/1 -> Estimated Velocity-to-be-gained/4(G_V_bar), [G_V_bar_mps2]
  Product9/1 -> Estimated Velocity-to-be-gained/2(V_V_bar), [V_V_bar_mps]
  Product8/1 -> [R_V_bar_m]
  XYZdotdot_VT_mps2/1 -> Estimated Velocity-to-be-gained/3(G_TV_bar)
  XYZdot_VT_mps/1 -> Estimated Velocity-to-be-gained/1(V_TV_bar)
  [tau_3_sec] -> Improved Estimate of Total time-to-go/2(tau_3_sec)
  [T_3_i_sec] -> Improved Estimate of Total time-to-go/1(T_3_i_sec), Add8/1
  Improved Estimate of Total time-to-go/1(Delta_T_prime_3) -> Add8/2, Product12/1
  [L_prime_y] -> Improved Estimate of Total time-to-go/4(L_prime_y)
  Add8/1 -> Data Store Write2/1, Add9/2, Position Correction Terms/3(T_3_i_sec)
  [T_1_i_sec] -> Add9/1, Position Correction Terms/6(T_1_i_sec)
  Product12/1 -> Add10/2
  Add10/1 -> Demux1/1, Vector Display2/1(In1)
  Demux1/1 -> Math Function1/1, Divide3/1
  Demux1/3 -> Math Function/1, Divide3/2
  Math Function/1 -> Add11/2
  Math Function1/1 -> Add11/1
  Add11/1 -> Math Function2/1
  Math Function2/1 -> Divide2/2
  Demux1/2 -> Divide2/1
  Divide2/1 -> Trigonometric Function3/1
  Divide3/1 -> Trigonometric Function4/1
  IGM Intermediate Parameters/2(J1) -> [J_1]
  IGM Intermediate Parameters/4(Q1) -> [Q_1]
  IGM Intermediate Parameters/5(P1) -> [P_1]
  IGM Intermediate Parameters/6(U1) -> [U_1]
  Trigonometric Function4/1 -> Position Correction Terms/18(Chi_y_tilde), Add12/1
  Trigonometric Function3/1 -> Position Correction Terms/17(Chi_z_tilde), Add14/1, Angle Conversion6/1
  [J_prime_3] -> Position Correction Terms/1(J_prime_3)
  [tau_3_sec] -> Position Correction Terms/2(tau_3_sec)
  [L_1] -> Position Correction Terms/4(L_1)
  [J_1] -> Position Correction Terms/5(J_1)
  [S_1] -> Position Correction Terms/7(S_1)
  [Q_1] -> Position Correction Terms/9(Q_1)
  [R_V_bar_m] -> Position Correction Terms/11(R_V_bar_m)
  [V_V_bar_mps] -> Position Correction Terms/12(V_V_bar_mps)
  [G_V_bar_mps2] -> Position Correction Terms/13(G_star_V_bar_mps2)
  Add9/1 -> Position Correction Terms/14(T_star)  "T_star"
  Improved Estimate of Total time-to-go/2(L_3) -> Position Correction Terms/15(L_3)
  Improved Estimate of Total time-to-go/3(Delta_L_3) -> Position Correction Terms/16(DeltaL_3)
  [P_1] -> Position Correction Terms/8(P_1)
  [U_1] -> Position Correction Terms/10(U_1)
  DeltaT_N_sec/1 -> Product13/2, Product14/2
  Position Correction Terms/2(K_2) -> Product13/1
  Product13/1 -> Add13/2
  Position Correction Terms/1(K_1) -> Add13/1
  [phi_T_rad] -> Add12/3
  const/1 -> Add12/4
  Product14/1 -> Add15/2
  Position Correction Terms/4(K_4) -> Product14/1
  Position Correction Terms/3(K_3) -> Add15/1
  Trigonometric Function2/1 -> Sum/1
  Sum1/1 -> Angle Conversion1/1
  Trigonometric Function5/1 -> Sum1/1
  Sum/1 -> Angle Conversion2/1
  Mux/1 -> Product15/2
  Product15/1 -> Demux2/1  "F_prime_S"
  Demux2/3 -> Unary Minus/1
  Demux2/1 -> Trigonometric Function5/2
  Constant7/1 -> Subtract/1
  Divide4/1 -> Trigonometric Function2/1
  Subtract/1 -> Math Function7/1
  Demux2/2 -> Math Function6/1, Divide4/1
  Math Function6/1 -> Subtract/2
  Math Function7/1 -> Divide4/2
  Math Function5/1 -> Product15/1
  [XYZdotdot_m_mps2] -> Demux3/1
  Add12/1 -> SinCos/1
  Add14/1 -> SinCos1/1, Angle Conversion5/1
  Product16/1 -> Mux/1
  SinCos/2 -> Product16/1
  SinCos1/2 -> Product16/2, Product17/2
  SinCos1/1 -> Mux/2
  Unary Minus1/1 -> Mux/3
  Product17/1 -> Unary Minus1/1
  SinCos/1 -> Product17/1
  [MS4] -> Math Function5/1
  Demux3/2 -> SMCZ/2(Ydotdot_m)
  [FoverM_mps2] -> SMCZ/3(FoverM)
  Constant10/1 -> MS4 Transform Matrix/1(A_z_deg)
  Constant11/1 -> MS4 Transform Matrix/2(phi_L_deg)
  Constant12/1 -> MS4 Transform Matrix/4(i_deg)
  Constant13/1 -> MS4 Transform Matrix/3(lambda_deg)
  G_S_bar_mps2/1 -> [G_S_bar_mps2]
  [T_star] -> Estimated Velocity-to-be-gained/5(T_star)
  [L_prime_3] -> Improved Estimate of Total time-to-go/5(L_prime_3)
  Mux1/1 -> Scope1/1
  Demux4/1 -> IGM Intermediate Parameters/1(tau_1_sec), Add1/1
  XYZdotdot_m_mps2/1 -> [XYZdotdot_m_mps2]
  Multiport Switch/1 -> Demux4/1
  Data Store Read2/1 -> Switch Case/1, Multiport Switch/1, Scope3/1
  IGM First Phase/1(tau_values) -> Multiport Switch/2
  IGM Phase2 (first BML)/1(tau_values) -> Multiport Switch/3
  IGM Phase2 (artificial tau mode)/1(tau_values) -> Multiport Switch/4
  IGM Phase2 (artificial tau complete)/1(tau_values) -> Multiport Switch/5
  Sum of Elements1/1 -> Math Function3/1
  Math Function4/1 -> Sum of Elements1/1
  Math Function3/1 -> [V], Memory1/1
  Switch Case/1 -> IGM First Phase/Action
  Switch Case/2 -> IGM Phase2 (first BML)/Action
  Switch Case/3 -> IGM Phase2 (artificial tau mode)/Action
  Switch Case/4 -> IGM Phase2 (artificial tau complete)/Action
  Product2/1 -> Add5/4
  T3_sec/1 -> [T3_sec]
  Demux3/1 -> SMCY/2(Xdotdot_m)
  Demux3/3 -> SMCY/3(Zdotdot_m)
  [G_star_V_bar] -> Product12/2
  Estimated Velocity-to-be-gained/2(G_star_V_bar) -> [G_star_V_bar]
  Estimated Velocity-to-be-gained/1(Delta_V_prime_V_bar) -> [Delta_V_prime_V_bar]
  [Delta_V_prime_V_bar] -> Improved Estimate of Total time-to-go/3(Delta_V_prime_V), Add10/1
  Angle Conversion1/1 -> IGM Chi Steering/1(Chi_Y)
  Add13/1 -> Add12/2
  Add15/1 -> Add14/2
  MF_S/1 -> IGM First Phase/1(MF_S), IGM Phase2 (artificial tau mode)/1(MF_S), IGM Phase2 (artificial tau complete)/1(MF_S), IGM Phase2 (first BML)/1(MF_S)
  Chi_minor_loop_sample/1 -> loop/1
  Selector1/1 -> Angle Conversion3/1
  Demux5/1 -> SMCY/1(Chi_y)
  Angle Conversion3/1 -> Demux5/1
  loop/1 -> Selector1/1
  Unary Minus/1 -> Trigonometric Function5/1
  Position Correction Terms/5(L_y) -> Terminator/1
  Position Correction Terms/6(C_2) -> Terminator1/1
  Position Correction Terms/7(C_4) -> Terminator2/1
  Angle Conversion2/1 -> +/- 45 degree limit/1, S-Frame Solution2/2
  Angle Conversion5/1 -> S-Frame Solution2/1
  Angle Conversion6/1 -> S-Frame Solution2/3
  Demux5/2 -> SMCZ/1(Chi_z)
  [T_3_i_sec] -> Compare To Constant2/1
  Compare To Constant2/1 -> DeltaT_b/Enable
  [V] -> DeltaT_b/1(V_mps)
  [V_prime] -> DeltaT_b/2(V_prime_mps)
  Switch Case/5 -> IGM Phase2 (HSL first pass)/Action
  IGM Phase2 (HSL first pass)/1(tau_values) -> Multiport Switch/6
  Memory1/1 -> Memory2/1, [V_prime]
  Memory2/1 -> [V_prime_prime]
  [V_prime] -> IGM Phase2 (HSL first pass)/2(V_prime_mps)
  [V_prime_prime] -> IGM Phase2 (HSL first pass)/3(V_prime_prime_mps)
  [V] -> IGM Phase2 (HSL first pass)/1(V_mps)
  Data Store Read1/1 -> Compare To Constant3/1
  HSL Cutoff Timing/1(bCutoff) -> bCutoff/1
  Compare To Constant3/1 -> HSL Cutoff Timing/Enable, Logical Operator1/1
  SMCY/1(SMCY_rad) -> Data Store Write/1
  SMCZ/1(SMCZ_rad) -> Data Store Write1/1
  Data Store Read/1 -> Sum1/2
  [T3_sec] -> Compare To Constant/1
  Compare To Constant/1 -> Logical Operator/2
  Logical Operator/1 -> [bSMCCalculate]
  Logical Operator1/1 -> Logical Operator/1
  Data Store Read3/1 -> Sum/2
  [bSMCCalculate] -> SMCZ/Enable, SMCY/Enable
  +/- 45 degree limit/1 -> IGM Chi Steering/2(Chi_Z)
  [T_3_i_sec] -> epsilon_prime/1
  epsilon_prime/1 -> IGM Chi Steering/Enable

== system saturn_ib_stack_test/Saturn_IB_Stack/Saturn Instrument Unit (IU)/LVDA / LVDC/LVDC S-Frame Position & Velocity Calculations ==
  note: V_m_bar represents the conditioned velocity accumulation
      | with a 0.05 m/s resolution.  This signal in this
      | model is equivalent to the output from
      | equation 4.2.8.
  note: "NASA Document says
      | 28.3608"
  note: per section 4.2.5 of EDD
  V_m_bar_mps : Inport  Port=1  LatchInput=off
  T3 : Inport  Port=2  SampleTime=1.6  LatchInput=off
  +/- 0.25 sec^2/m : Saturate  UpperLimit=4.00  LowerLimit=-4.00
  Az_deg : Constant  Value=A_z_deg
  Constant4 : Constant  Value=delta_T_sec  OutDataTypeMode=double
  Constant5 : Constant  Value=0.0  OutDataTypeMode=double
  Estimated Gravitational Acceleration (Eqns. 4.3.6-12) : Subsystem  mask{a_e_m=6378165.0, b_m=6356783.0, D=0.7875E-05, H=0.575E-05, J=1.62345E-03, mu=3.986032E+14}
      mask prompts: a_e_m "a_e"; b_m "b"; mu "mu (m^3/sec^2)"
  Initial Position and Velocity (Eqns. 3.4.3-4) : Subsystem  mask{omega_E_rps=0.000023211523}
  Position and Velocity Calculation (S-Frame) (Eqns. 4.3.1-5) : Subsystem
  R_L : Constant  Value=R_L_m
  Rate Limiter +/- 0.005 : RateLimiter  RisingSlewLimit=0.005  FallingSlewLimit=-0.005  SampleTimeMode=inherited
  Reciprocal Acceleration Filter (EDD eqn. 4.2.11) : Subsystem
  T3_FM : simulink/Logic and Bit Operations/Compare To Constant  relop=>=  const=T3_FM_sec  LogicOutDataTypeMode=uint8  ZeroCross=off
  Terminator : Terminator
  phi_L_deg : Constant  Value=phi_L_deg
  phi_L_prime_deg : Constant  Value=phi_L_prime_deg
  R_S_bar_m : Outport
  V_S_bar_mps : Outport  Port=2
  G_S_bar_mps2 : Outport  Port=3
  A_m_bar_mps2 : Outport  Port=4
  FoverM_mps2 : Outport  Port=5
  MoverF_S : Outport  Port=6
  wires:
  Estimated Gravitational Acceleration (Eqns. 4.3.6-12)/2(G_S_bar_mps2) -> G_S_bar_mps2/1, Position and Velocity Calculation (S-Frame) (Eqns. 4.3.1-5)/2(XYZdotdot_Sg_mps2)
  Constant4/1 -> Position and Velocity Calculation (S-Frame) (Eqns. 4.3.1-5)/5(Delta_T_sec)
  Az_deg/1 -> Estimated Gravitational Acceleration (Eqns. 4.3.6-12)/2(A_z_deg), Initial Position and Velocity (Eqns. 3.4.3-4)/2(A_z_deg)
  phi_L_deg/1 -> Estimated Gravitational Acceleration (Eqns. 4.3.6-12)/3(phi_L_deg), Initial Position and Velocity (Eqns. 3.4.3-4)/3(phi_L_deg)
  Initial Position and Velocity (Eqns. 3.4.3-4)/2(V_S_0_mps) -> Position and Velocity Calculation (S-Frame) (Eqns. 4.3.1-5)/4(XYZdot_0_mps)
  R_L/1 -> Initial Position and Velocity (Eqns. 3.4.3-4)/1(R_L_m)
  phi_L_prime_deg/1 -> Initial Position and Velocity (Eqns. 3.4.3-4)/4(phi_L_prime_deg)
  Constant5/1 -> Position and Velocity Calculation (S-Frame) (Eqns. 4.3.1-5)/6(TGRR_bias_sec)
  Initial Position and Velocity (Eqns. 3.4.3-4)/1(R_S_0_m) -> Position and Velocity Calculation (S-Frame) (Eqns. 4.3.1-5)/3(XYZ_0_m)
  Estimated Gravitational Acceleration (Eqns. 4.3.6-12)/1(Y_G_m) -> Terminator/1
  Position and Velocity Calculation (S-Frame) (Eqns. 4.3.1-5)/1(XYZ_S_m) -> R_S_bar_m/1, Estimated Gravitational Acceleration (Eqns. 4.3.6-12)/1(XYZ_S_m)
  V_m_bar_mps/1 -> Position and Velocity Calculation (S-Frame) (Eqns. 4.3.1-5)/1(XYZdot_m_mps)
  Position and Velocity Calculation (S-Frame) (Eqns. 4.3.1-5)/2(XYZdot_S_mps) -> V_S_bar_mps/1
  Position and Velocity Calculation (S-Frame) (Eqns. 4.3.1-5)/3(A_m_bar_mps2) -> A_m_bar_mps2/1
  Position and Velocity Calculation (S-Frame) (Eqns. 4.3.1-5)/4(FoverM_mps2) -> FoverM_mps2/1, Reciprocal Acceleration Filter (EDD eqn. 4.2.11)/1(A_S_mps2)
  Reciprocal Acceleration Filter (EDD eqn. 4.2.11)/1(MF_S) -> +/- 0.25 sec^2/m/1
  Rate Limiter +/- 0.005/1 -> MoverF_S/1
  T3/1 -> T3_FM/1
  T3_FM/1 -> Reciprocal Acceleration Filter (EDD eqn. 4.2.11)/Enable
  +/- 0.25 sec^2/m/1 -> Rate Limiter +/- 0.005/1

== system saturn_ib_stack_test/Saturn_IB_Stack/Saturn Instrument Unit (IU)/LVDA / LVDC/T1 Timer ==
  bStart : Inport  Port=1  DataType=boolean  LatchInput=off
  Clock : Clock
      settings: Decimation=10
  Constant : Constant  Value=0.0
  Data Store Memory : DataStoreMemory  DataStoreName=A  InitialValue=-1  DataType=double
  Data Store Read : DataStoreRead  DataStoreName=A  SampleTime=0
  Sum : Sum  Inputs=|+-
  Switch : Switch  Threshold=0.0
  Timer Initialization : Subsystem  TreatAsAtomicUnit=on
  T_elapsed_sec : Outport
  wires:
  bStart/1 -> Timer Initialization/Trigger
  Clock/1 -> Timer Initialization/1(In1), Sum/1
  Switch/1 -> T_elapsed_sec/1
  Sum/1 -> Switch/1
  Data Store Read/1 -> Sum/2, Switch/2
  Constant/1 -> Switch/3

== system saturn_ib_stack_test/Saturn_IB_Stack/Saturn Instrument Unit (IU)/LVDA / LVDC/T2 Timer ==
  bStart : Inport  Port=1  DataType=boolean  LatchInput=off
  Clock : Clock
      settings: Decimation=10
  Constant : Constant  Value=0.0
  Data Store Memory : DataStoreMemory  DataStoreName=A  InitialValue=-1  DataType=double
  Data Store Read : DataStoreRead  DataStoreName=A  SampleTime=0
  Sum : Sum  Inputs=|+-
  Switch : Switch  Threshold=0.0
  Timer Initialization : Subsystem  TreatAsAtomicUnit=on
  T_elapsed_sec : Outport
  wires:
  bStart/1 -> Timer Initialization/Trigger
  Clock/1 -> Timer Initialization/1(In1), Sum/1
  Switch/1 -> T_elapsed_sec/1
  Sum/1 -> Switch/1
  Data Store Read/1 -> Sum/2, Switch/2
  Constant/1 -> Switch/3

== system saturn_ib_stack_test/Saturn_IB_Stack/Saturn Instrument Unit (IU)/LVDA / LVDC/T3 Timer ==
  bStart : Inport  Port=1  DataType=boolean  LatchInput=off
  Clock : Clock
      settings: Decimation=10
  Constant : Constant  Value=0.0
  Data Store Memory : DataStoreMemory  DataStoreName=A  InitialValue=-1  DataType=double
  Data Store Read : DataStoreRead  DataStoreName=A  SampleTime=0
  Sum : Sum  Inputs=|+-
  Switch : Switch  Threshold=0.0
  Timer Initialization : Subsystem  TreatAsAtomicUnit=on
  T_elapsed_sec : Outport
  wires:
  bStart/1 -> Timer Initialization/Trigger
  Clock/1 -> Timer Initialization/1(In1), Sum/1
  Switch/1 -> T_elapsed_sec/1
  Sum/1 -> Switch/1
  Data Store Read/1 -> Sum/2, Switch/2
  Constant/1 -> Switch/3
